simulink library "control_command_generation_lib"  (R2018b)
settings: Solver=VariableStepAuto  StartTime=0.0  StopTime=10.0  RelTol=1e-3
undefined symbols (not defined in the file): fswParams
libraries: aerolibutil x2, Desat_Controller_Logic_lib x1, SlewAndControlConstrained_Controller_lib x1, PD_Controller_Lib x1, Detumbling_Controller_lib x1, Desaturation_Controller_lib x1, command_converter_lib x1
settings Model: Creator=colem  LastModifiedBy=colem

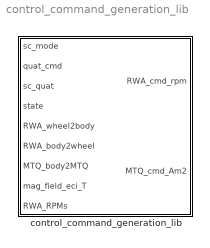
== system control_command_generation_lib ==
  control_command_generation_lib : Subsystem

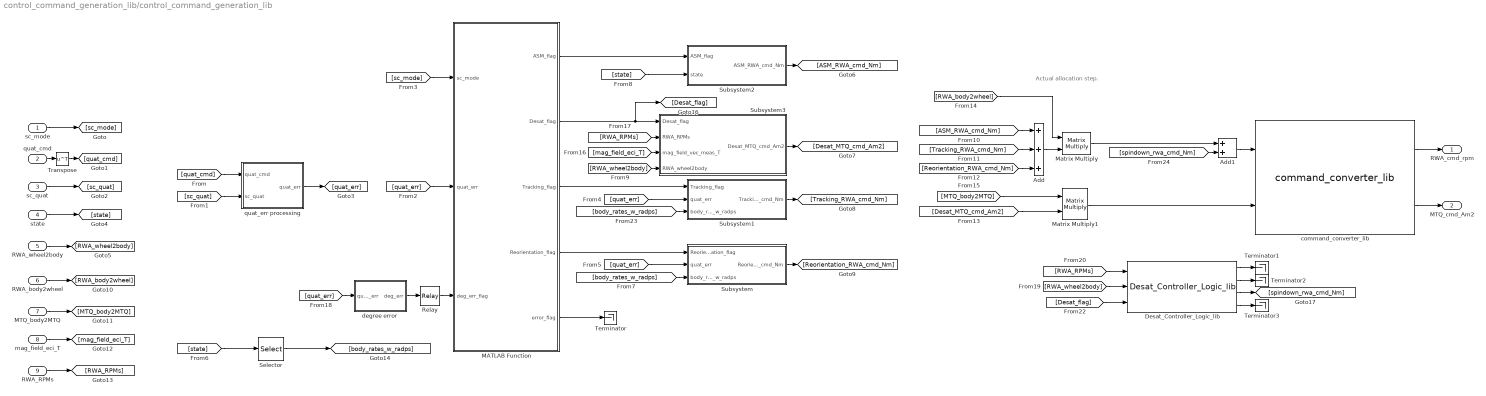
== system control_command_generation_lib/control_command_generation_lib ==
  note: Actual allocation step.
  sc_mode : Inport
  quat_cmd : Inport  Port=2
  sc_quat : Inport  Port=3
  state : Inport  Port=4
  RWA_wheel2body : Inport  Port=5
  RWA_body2wheel : Inport  Port=6
  MTQ_body2MTQ : Inport  Port=7
  mag_field_eci_T : Inport  Port=8
  RWA_RPMs : Inport  Port=9
  Add : Sum  Inputs=3
  Add1 : Sum
  Desat_Controller_Logic_lib : Desat_Controller_Logic_lib/Desat_Controller_Logic_lib  SystemSampleTime=-1
  MATLAB Function : MATLAB Function  TreatAsAtomicUnit=on
  Matrix Multiply : Product  Multiplication=Matrix(*)
  Matrix Multiply1 : Product  Multiplication=Matrix(*)
  Relay : Relay  OnSwitchValue=fswParams.constants.global.reorientation_controller_threshold_max  OffSwitchValue=fswParams.constants.global.reorientation_controller_threshold_max
  Selector : Selector  InputPortWidth=13  IndexOptions=Index vector (dialog)  Indices=[11 12 13]  OutputSizes=1
  Subsystem : Subsystem
  Subsystem1 : Subsystem
  Subsystem2 : Subsystem
  Subsystem3 : Subsystem
  Terminator{,1..3} (4 alike) : Terminator
  Transpose : Math  Operator=transpose  SaturateOnIntegerOverflow=on
  command_converter_lib : command_converter_lib/command_converter_lib  SystemSampleTime=-1
  degree error : Subsystem
  quat_err processing : Subsystem
  RWA_cmd_rpm : Outport
  MTQ_cmd_Am2 : Outport  Port=2
  wires:
  sc_mode/1 -> [sc_mode]
  quat_cmd/1 -> Transpose/1
  sc_quat/1 -> [sc_quat]
  [quat_err] -> MATLAB Function/2(quat_err)
  [sc_mode] -> MATLAB Function/1(sc_mode)
  MATLAB Function/5(error_flag) -> Terminator/1
  [quat_err] -> Subsystem/2(quat_err)
  [body_rates_w_radps] -> Subsystem/3(body_rates_w_radps)
  Subsystem/1(Reorient_RWA_cmd_Nm) -> [Reorientation_RWA_cmd_Nm]
  state/1 -> [state]
  [quat_err] -> Subsystem1/2(quat_err)
  [body_rates_w_radps] -> Subsystem1/3(body_rates_w_radps)
  [state] -> Subsystem2/2(state)
  MATLAB Function/1(ASM_flag) -> Subsystem2/1(ASM_flag)
  MATLAB Function/2(Desat_flag) -> [Desat_flag], Subsystem3/1(Desat_flag)
  RWA_wheel2body/1 -> [RWA_wheel2body]
  [RWA_wheel2body] -> Subsystem3/4(RWA_wheel2body)
  Subsystem2/1(ASM_RWA_cmd_Nm) -> [ASM_RWA_cmd_Nm]
  Subsystem1/1(Tracking_RWA_cmd_Nm) -> [Tracking_RWA_cmd_Nm]
  [ASM_RWA_cmd_Nm] -> Add/1
  [Tracking_RWA_cmd_Nm] -> Add/2
  [Reorientation_RWA_cmd_Nm] -> Add/3
  Add/1 -> Matrix Multiply/2
  [Desat_MTQ_cmd_Am2] -> Matrix Multiply1/2
  command_converter_lib/2 -> MTQ_cmd_Am2/1
  RWA_body2wheel/1 -> [RWA_body2wheel]
  [RWA_body2wheel] -> Matrix Multiply/1
  Matrix Multiply/1 -> Add1/1
  MTQ_body2MTQ/1 -> [MTQ_body2MTQ]
  [MTQ_body2MTQ] -> Matrix Multiply1/1
  Matrix Multiply1/1 -> command_converter_lib/2
  mag_field_eci_T/1 -> [mag_field_eci_T]
  RWA_RPMs/1 -> [RWA_RPMs]
  [mag_field_eci_T] -> Subsystem3/3(mag_field_vec_meas_T)
  Transpose/1 -> [quat_cmd]
  MATLAB Function/3(Tracking_flag) -> Subsystem1/1(Tracking_flag)
  MATLAB Function/4(Reorientation_flag) -> Subsystem/1(Reorientation_flag)
  Subsystem3/1(Desat_MTQ_cmd_Am2) -> [Desat_MTQ_cmd_Am2]
  [RWA_RPMs] -> Subsystem3/2(RWA_RPMs)
  [quat_err] -> degree error/1(quat_err)
  degree error/1(deg_err) -> Relay/1
  Relay/1 -> MATLAB Function/3(deg_err_flag)
  [RWA_wheel2body] -> Desat_Controller_Logic_lib/2
  [RWA_RPMs] -> Desat_Controller_Logic_lib/1
  Desat_Controller_Logic_lib/1 -> Terminator1/1
  Desat_Controller_Logic_lib/3 -> [spindown_rwa_cmd_Nm]
  Desat_Controller_Logic_lib/2 -> Terminator2/1
  [Desat_flag] -> Desat_Controller_Logic_lib/3
  command_converter_lib/1 -> RWA_cmd_rpm/1
  [quat_cmd] -> quat_err processing/1(quat_cmd)
  [sc_quat] -> quat_err processing/2(sc_quat)
  quat_err processing/1(quat_err) -> [quat_err]
  [state] -> Selector/1
  Selector/1 -> [body_rates_w_radps]
  Desat_Controller_Logic_lib/4 -> Terminator3/1
  [spindown_rwa_cmd_Nm] -> Add1/2
  Add1/1 -> command_converter_lib/1

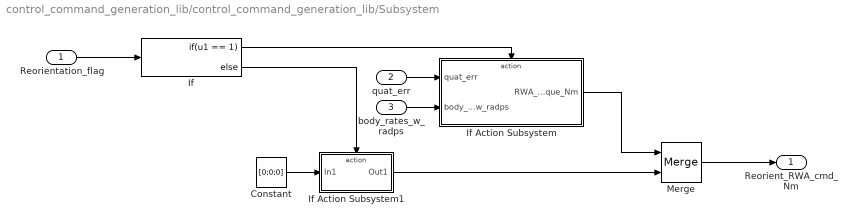
== system control_command_generation_lib/control_command_generation_lib/Subsystem ==
  Reorientation_flag : Inport
  quat_err : Inport  Port=2
  body_rates_w_radps : Inport  Port=3
  Constant : Constant  Value=[0;0;0]
  If : If  IfExpression=u1 == 1
  If Action Subsystem : Subsystem  TreatAsAtomicUnit=on
  If Action Subsystem1 : Subsystem  TreatAsAtomicUnit=on
  Merge : Merge
  Reorient_RWA_cmd_Nm : Outport
  wires:
  quat_err/1 -> If Action Subsystem/1(quat_err)
  Merge/1 -> Reorient_RWA_cmd_Nm/1
  If Action Subsystem1/1(Out1) -> Merge/2
  body_rates_w_radps/1 -> If Action Subsystem/2(body_rates_w_radps)
  If Action Subsystem/1(RWA_cmd_torque_Nm) -> Merge/1
  If/2 -> If Action Subsystem1/Action
  Reorientation_flag/1 -> If/1
  Constant/1 -> If Action Subsystem1/1(In1)
  If/1 -> If Action Subsystem/Action

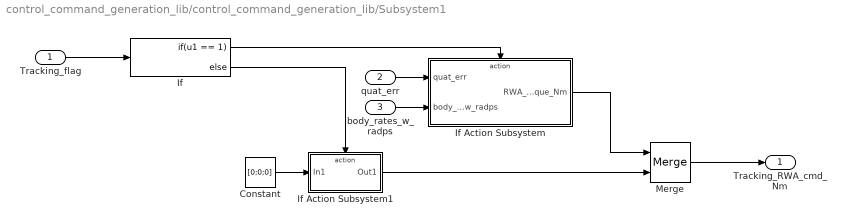
== system control_command_generation_lib/control_command_generation_lib/Subsystem1 ==
  Tracking_flag : Inport
  quat_err : Inport  Port=2
  body_rates_w_radps : Inport  Port=3
  Constant : Constant  Value=[0;0;0]
  If : If  IfExpression=u1 == 1
  If Action Subsystem : Subsystem  TreatAsAtomicUnit=on
  If Action Subsystem1 : Subsystem  TreatAsAtomicUnit=on
  Merge : Merge
  Tracking_RWA_cmd_Nm : Outport
  wires:
  quat_err/1 -> If Action Subsystem/1(quat_err)
  Merge/1 -> Tracking_RWA_cmd_Nm/1
  If Action Subsystem1/1(Out1) -> Merge/2
  body_rates_w_radps/1 -> If Action Subsystem/2(body_rates_w_radps)
  If Action Subsystem/1(RWA_cmd_torque_Nm) -> Merge/1
  If/2 -> If Action Subsystem1/Action
  Tracking_flag/1 -> If/1
  Constant/1 -> If Action Subsystem1/1(In1)
  If/1 -> If Action Subsystem/Action

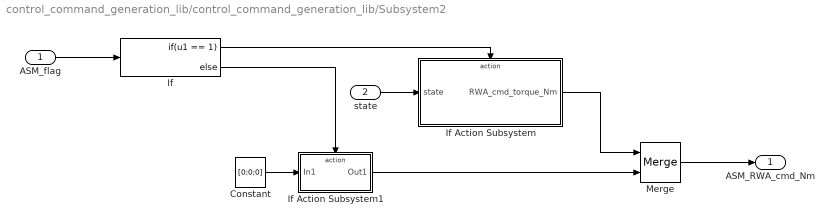
== system control_command_generation_lib/control_command_generation_lib/Subsystem2 ==
  ASM_flag : Inport
  state : Inport  Port=2
  Constant : Constant  Value=[0;0;0]
  If : If  IfExpression=u1 == 1
  If Action Subsystem : Subsystem  TreatAsAtomicUnit=on
  If Action Subsystem1 : Subsystem  TreatAsAtomicUnit=on
  Merge : Merge
  ASM_RWA_cmd_Nm : Outport
  wires:
  Merge/1 -> ASM_RWA_cmd_Nm/1
  If Action Subsystem1/1(Out1) -> Merge/2
  state/1 -> If Action Subsystem/1(state)
  If Action Subsystem/1(RWA_cmd_torque_Nm) -> Merge/1
  If/2 -> If Action Subsystem1/Action
  ASM_flag/1 -> If/1
  Constant/1 -> If Action Subsystem1/1(In1)
  If/1 -> If Action Subsystem/Action

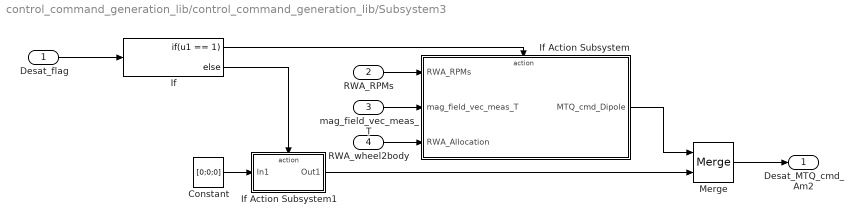
== system control_command_generation_lib/control_command_generation_lib/Subsystem3 ==
  Desat_flag : Inport
  RWA_RPMs : Inport  Port=2
  mag_field_vec_meas_T : Inport  Port=3
  RWA_wheel2body : Inport  Port=4
  Constant : Constant  Value=[0;0;0]
  If : If  IfExpression=u1 == 1
  If Action Subsystem : Subsystem  TreatAsAtomicUnit=on
  If Action Subsystem1 : Subsystem  TreatAsAtomicUnit=on
  Merge : Merge
  Desat_MTQ_cmd_Am2 : Outport
  wires:
  Merge/1 -> Desat_MTQ_cmd_Am2/1
  If Action Subsystem1/1(Out1) -> Merge/2
  RWA_RPMs/1 -> If Action Subsystem/1(RWA_RPMs)
  If Action Subsystem/1(MTQ_cmd_Dipole) -> Merge/1
  If/2 -> If Action Subsystem1/Action
  Desat_flag/1 -> If/1
  Constant/1 -> If Action Subsystem1/1(In1)
  If/1 -> If Action Subsystem/Action
  mag_field_vec_meas_T/1 -> If Action Subsystem/2(mag_field_vec_meas_T)
  RWA_wheel2body/1 -> If Action Subsystem/3(RWA_Allocation)

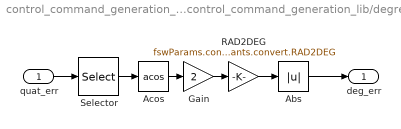
== system control_command_generation_lib/control_command_generation_lib/degree error ==
  quat_err : Inport
  Abs : Abs
  Acos : Trigonometry  Operator=acos
  Gain : Gain  Gain=2
  RAD2DEG : Gain  Gain=fswParams.constants.convert.RAD2DEG
  Selector : Selector  InputPortWidth=4  IndexOptions=Index vector (dialog)  Indices=[1]  OutputSizes=1
  deg_err : Outport
  wires:
  RAD2DEG/1 -> Abs/1
  Gain/1 -> RAD2DEG/1
  Acos/1 -> Gain/1
  Selector/1 -> Acos/1
  Abs/1 -> deg_err/1
  quat_err/1 -> Selector/1

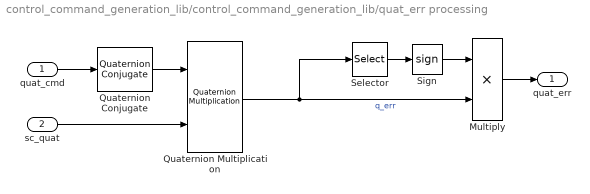
== system control_command_generation_lib/control_command_generation_lib/quat_err processing ==
  quat_cmd : Inport
  sc_quat : Inport  Port=2
  Multiply : Product
  Quaternion Conjugate : aerolibutil/Quaternion Conjugate
      settings: SourceProductName=Aerospace Blockset  SourceProductBaseCode=AE
  Quaternion Multiplication : aerolibutil/Quaternion Multiplication
  Selector : Selector  InputPortWidth=4  IndexOptions=Index vector (dialog)  Indices=[1]  OutputSizes=1
  Sign : Signum
  quat_err : Outport
  wires:
  Quaternion Multiplication/1 -> Multiply/2, Selector/1  "q_err"
  Quaternion Conjugate/1 -> Quaternion Multiplication/1
  Sign/1 -> Multiply/1
  Selector/1 -> Sign/1
  sc_quat/1 -> Quaternion Multiplication/2
  Multiply/1 -> quat_err/1
  quat_cmd/1 -> Quaternion Conjugate/1

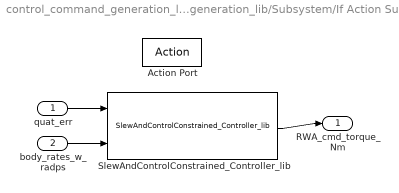
== system control_command_generation_lib/control_command_generation_lib/Subsystem/If Action Subsystem ==
  quat_err : Inport
  body_rates_w_radps : Inport  Port=2
  Action Port : ActionPort  ActionType=then
  SlewAndControlConstrained_Controller_lib : SlewAndControlConstrained_Controller_lib/SlewAndControlConstrained_Controller_lib  SystemSampleTime=-1
  RWA_cmd_torque_Nm : Outport
  wires:
  quat_err/1 -> SlewAndControlConstrained_Controller_lib/1
  body_rates_w_radps/1 -> SlewAndControlConstrained_Controller_lib/2
  SlewAndControlConstrained_Controller_lib/1 -> RWA_cmd_torque_Nm/1

== system control_command_generation_lib/control_command_generation_lib/Subsystem/If Action Subsystem1 ==
  In1 : Inport
  Action Port : ActionPort  ActionType=else
  Out1 : Outport
  wires:
  In1/1 -> Out1/1

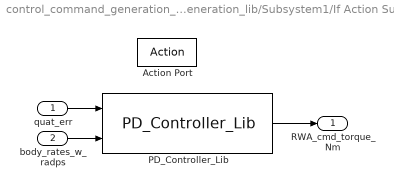
== system control_command_generation_lib/control_command_generation_lib/Subsystem1/If Action Subsystem ==
  quat_err : Inport
  body_rates_w_radps : Inport  Port=2
  Action Port : ActionPort
  PD_Controller_Lib : PD_Controller_Lib/PD_Controller_Lib  SystemSampleTime=-1
  RWA_cmd_torque_Nm : Outport
  wires:
  quat_err/1 -> PD_Controller_Lib/1
  body_rates_w_radps/1 -> PD_Controller_Lib/2
  PD_Controller_Lib/1 -> RWA_cmd_torque_Nm/1

== system control_command_generation_lib/control_command_generation_lib/Subsystem1/If Action Subsystem1 ==
  In1 : Inport
  Action Port : ActionPort
  Out1 : Outport
  wires:
  In1/1 -> Out1/1

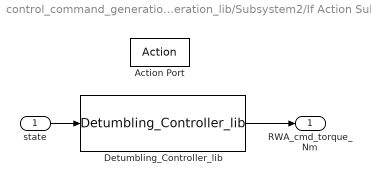
== system control_command_generation_lib/control_command_generation_lib/Subsystem2/If Action Subsystem ==
  state : Inport
  Action Port : ActionPort
  Detumbling_Controller_lib : Detumbling_Controller_lib/Detumbling_Controller_lib  SystemSampleTime=-1
  RWA_cmd_torque_Nm : Outport
  wires:
  state/1 -> Detumbling_Controller_lib/1
  Detumbling_Controller_lib/1 -> RWA_cmd_torque_Nm/1

== system control_command_generation_lib/control_command_generation_lib/Subsystem2/If Action Subsystem1 ==
  In1 : Inport
  Action Port : ActionPort
  Out1 : Outport
  wires:
  In1/1 -> Out1/1

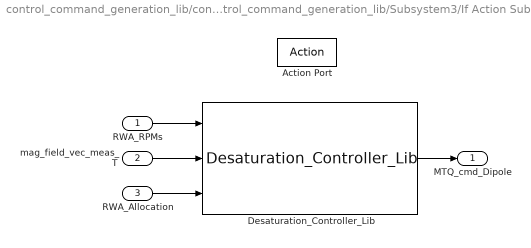
== system control_command_generation_lib/control_command_generation_lib/Subsystem3/If Action Subsystem ==
  RWA_RPMs : Inport
  mag_field_vec_meas_T : Inport  Port=2
  RWA_Allocation : Inport  Port=3
  Action Port : ActionPort
  Desaturation_Controller_Lib : Desaturation_Controller_lib/Desaturation_Controller_Lib  SystemSampleTime=-1
  MTQ_cmd_Dipole : Outport
  wires:
  RWA_RPMs/1 -> Desaturation_Controller_Lib/1
  Desaturation_Controller_Lib/1 -> MTQ_cmd_Dipole/1
  mag_field_vec_meas_T/1 -> Desaturation_Controller_Lib/2
  RWA_Allocation/1 -> Desaturation_Controller_Lib/3

== system control_command_generation_lib/control_command_generation_lib/Subsystem3/If Action Subsystem1 ==
  In1 : Inport
  Action Port : ActionPort
  Out1 : Outport
  wires:
  In1/1 -> Out1/1

== matlab function control_command_generation_lib/MATLAB Function ==
  data: sc_mode input; ASM_flag output; quat_err input; Desat_flag output; Tracking_flag output; Reorientation_flag output; error_flag output; deg_err_flag input
% Logic for selecting the gnc control mode. Based on the sc mode, the
% control scheme is selected.
%
% Author: Cole Morgan 11.07.19
%
% 



function [ASM_flag, Desat_flag, Tracking_flag, Reorientation_flag, error_flag]...
                                        = control_selection_logic(sc_mode, quat_err, deg_err_flag)

%GNC_MODE_LOGIC    GNC sc modes
%
% Chooses controller based on sc mode.
%   mode_logic.low_power        = 1; "safe mode"
%   mode_logic.idle             = 2; "idle/standby mode"
%   mode_logic.stabilize        = 3;
%   mode_logic.nominal          = 4;
%       nominal.desat           = 41;
%       nominal.sun_seek        = 42;
%   mode_logic.point            = 5;
%       point.com               = 51;
%       point.image             = 52;
%       point.exp               = 53;
%
% ----- INPUTS -----
% 
% sc_mode - modes outlined above.
%
% quat_err - error between current and commanded attitude.
%
% ----- OUTPUTS -----
%
% ASM_flag - flag turning Attitude Stabilization (Detumble) controller on/off 
% Desat_flag - flag turning Desaturation controller on/off
% Tracking_flag - flag turning Tracking controller on/off 
% Reorientation_flag - flag turning Large-angle Reorientation controller on/off
% error_flag - indicates this function has failed to find a control scheme
%       when it should have found one.



% Default to no controller selection and some error meaning you didn't ever even trip it.
ASM_flag           = 0;
Desat_flag         = 0;
Tracking_flag      = 0;
Reorientation_flag = 0; 
error_flag         = -1;

% quat_err indicates if large angle reorientation 
% is necessary.
% deg_err is the total error in degrees from the desired
% orientation. If this value is not small, use (or keep using) 
% large-angle reorientation controller until it is small enough to track.
% deg_err = abs(2*acosd(quat_err(1)));

% If sc_mode is not LPM or CLPM
if( sc_mode ~= 1.0 && sc_mode ~= 2.0)
    error_flag = 0;
    
    % engage ASM controller
    if (sc_mode == 3.0)
        ASM_flag = 1;
        
    % engage Desat controller, but Tracking
    % must be maintained.
    elseif (sc_mode == 41.0)
        Desat_flag = 1;
%         Tracking_flag = 1;
        ASM_flag = 1;
        return;
        
    % engage (or keep) Tracking controller engaged in any mode with an  
    % attitude objective. This is the most likely scenario.
    elseif (sc_mode == 42.0 || sc_mode == 51.0 || sc_mode == 52.0 || sc_mode == 53.0)
        Tracking_flag = 1;
        
        % If the angular error is larger than the threshold set in fswParams,
        % (typically less than 3.5 degrees) then a large angle reorientation 
        % is needed.
        if (deg_err_flag) %>= reorientation_controller_threshold)
            Reorientation_flag = 1;
            Tracking_flag = 0;
        end
        
    else
        % indicates we are not in LPM or CLPM and still
        % are not getting a control scheme correctly.
        error_flag = 1;
    end
    
    % Final protection from asking for multiple RWA control schemes.
    % If so, just keep attitude stable.
    check = ASM_flag + Tracking_flag + Reorientation_flag;
    if (check > 1)
        ASM_flag = 1;
        Tracking_flag = 0;
        Reorientation_flag = 0;
        error_flag = 2;
    end
    
    
end
